simulink model "Linearisierung3_Robo_Sim"  (R2017a)
settings: Solver=VariableStepAuto  StartTime=0.0  StopTime=10.0  RelTol=1e-3
values from neighbouring files (symbols this model uses):
  c = 1    [Linearisierung3_Robo.m]
  g = 9.81    [Linearisierung3_Robo.m]
  l = 1    [Linearisierung3_Robo.m]
  m = 7    [Linearisierung3_Robo.m]
settings Model: Creator=Jonas  LastModifiedBy=Jonas

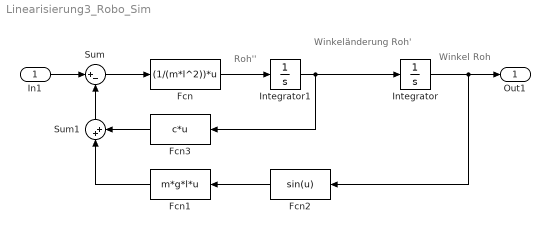
== system Linearisierung3_Robo_Sim ==
  note: Roh''
  note: Winkeländerung
      | Roh'
  note: Winkel Roh
  In1 : Inport
  Fcn : Fcn  Expr=(1/(m*l^2))*u
  Fcn1 : Fcn  Expr=m*g*l*u
  Fcn2 : Fcn  Expr=sin(u)
  Fcn3 : Fcn  Expr=c*u
  Integrator : Integrator
  Integrator1 : Integrator
  Sum : Sum  Inputs=|+-
  Sum1 : Sum  Inputs=|++
  Out1 : Outport
  wires:
  Sum1/1 -> Sum/2
  In1/1 -> Sum/1
  Sum/1 -> Fcn/1
  Fcn3/1 -> Sum1/2
  Fcn1/1 -> Sum1/1
  Fcn2/1 -> Fcn1/1
  Integrator/1 -> Fcn2/1, Out1/1
  Integrator1/1 -> Fcn3/1, Integrator/1
  Fcn/1 -> Integrator1/1
